simulink model "plant"  (R2026a)
settings: Solver=VariableStepAuto  StopTime=11
InitFcn:
  | run('plant_parameters.m');
values from neighbouring files (symbols this model uses):
  d = 0.1845    [plant_parameters.m]
  dd = d / sqrt(2)    [plant_parameters.m]
  Kd_J1 = 40    [plant_parameters.m]
  Kd_J2 = 30    [plant_parameters.m]
  Kd_J3 = 12    [plant_parameters.m]
  Ki_J1 = 800    [plant_parameters.m]
  Ki_J2 = 700    [plant_parameters.m]
  Ki_J3 = 300    [plant_parameters.m]
  Kp_J1 = 800    [plant_parameters.m]
  Kp_J2 = 600    [plant_parameters.m]
  Kp_J3 = 250    [plant_parameters.m]
  L1 = 0.074    [plant_parameters.m]
  L2 = 0.121    [plant_parameters.m]
  L3 = 0.230    (= 0.23)    [plant_parameters.m]
  N_J1 = 120    [plant_parameters.m]
  N_J2 = 120    [plant_parameters.m]
  N_J3 = 120    [plant_parameters.m]
  Sampling_Time = 0.005    [plant_parameters.m]
undefined symbols (not defined in the file or in its folder): X, Y, Z
libraries: sm_lib x121, nesl_utility x55, slpidlib x18
(part 8 of 8)

== matlab function plant/MATLAB Function26 ==
  data: xB_1 input; Body_X_Est output; yB_1 input; zB_1 input; xB_2 input; yB_2 input; zB_2 input; xB_3 input; yB_3 input; zB_3 input; xB_4 input; yB_4 input; zB_4 input; xB_5 input; yB_5 input; zB_5 input; xB_6 input; yB_6 input; zB_6 input; Leg1_State input; Leg2_State input; Leg3_State input; Leg4_State input; Leg5_State input; Leg6_State input; Contact6 input; Contact5 input; Contact4 input; Contact3 input; Contact2 input; Contact1 input; Body_Y_Est output; Body_Z_Est output; Valid_Leg_Count output
% Stance Contact 발의 FK 위치로 몸체 위치를 추정한다.
function [Body_X_Est, Body_Y_Est, Body_Z_Est, ...
          Valid_Leg_Count] = BodyPositionEstimator( ...
          xB_1, yB_1, zB_1, ...
          xB_2, yB_2, zB_2, ...
          xB_3, yB_3, zB_3, ...
          xB_4, yB_4, zB_4, ...
          xB_5, yB_5, zB_5, ...
          xB_6, yB_6, zB_6, ...
          Leg1_State, Leg2_State, Leg3_State, ...
          Leg4_State, Leg5_State, Leg6_State, ...
          Contact6, Contact5, Contact4, ...
          Contact3, Contact2, Contact1)

STANCE = 0;  % Stance 상태 번호를 정의한다.

persistent Initialized
persistent Body_X_Memory Body_Y_Memory Body_Z_Memory

persistent Anchor_X_1 Anchor_Y_1 Anchor_Z_1 Was_Valid_1
persistent Anchor_X_2 Anchor_Y_2 Anchor_Z_2 Was_Valid_2
persistent Anchor_X_3 Anchor_Y_3 Anchor_Z_3 Was_Valid_3
persistent Anchor_X_4 Anchor_Y_4 Anchor_Z_4 Was_Valid_4
persistent Anchor_X_5 Anchor_Y_5 Anchor_Z_5 Was_Valid_5
persistent Anchor_X_6 Anchor_Y_6 Anchor_Z_6 Was_Valid_6

% 최초 실행 시 추정 위치와 Anchor를 초기화한다.
if isempty(Initialized)
    Initialized = true;

    Body_X_Memory = 0;
    Body_Y_Memory = 0;
    Body_Z_Memory = 0;

    Anchor_X_1 = 0;
    Anchor_Y_1 = 0;
    Anchor_Z_1 = 0;
    Was_Valid_1 = false;

    Anchor_X_2 = 0;
    Anchor_Y_2 = 0;
    Anchor_Z_2 = 0;
    Was_Valid_2 = false;

    Anchor_X_3 = 0;
    Anchor_Y_3 = 0;
    Anchor_Z_3 = 0;
    Was_Valid_3 = false;

    Anchor_X_4 = 0;
    Anchor_Y_4 = 0;
    Anchor_Z_4 = 0;
    Was_Valid_4 = false;

    Anchor_X_5 = 0;
    Anchor_Y_5 = 0;
    Anchor_Z_5 = 0;
    Was_Valid_5 = false;

    Anchor_X_6 = 0;
    Anchor_Y_6 = 0;
    Anchor_Z_6 = 0;
    Was_Valid_6 = false;
end

% 1번 다리의 Anchor와 몸체 위치 후보를 계산한다.
[Anchor_X_1, Anchor_Y_1, Anchor_Z_1, Was_Valid_1, ...
 Valid_1, Body_X_1, Body_Y_1, Body_Z_1] = UpdateLegEstimate( ...
    xB_1, yB_1, zB_1, Leg1_State, Contact1, ...
    Anchor_X_1, Anchor_Y_1, Anchor_Z_1, Was_Valid_1, ...
    Body_X_Memory, Body_Y_Memory, Body_Z_Memory, STANCE);

% 2번 다리의 Anchor와 몸체 위치 후보를 계산한다.
[Anchor_X_2, Anchor_Y_2, Anchor_Z_2, Was_Valid_2, ...
 Valid_2, Body_X_2, Body_Y_2, Body_Z_2] = UpdateLegEstimate( ...
    xB_2, yB_2, zB_2, Leg2_State, Contact2, ...
    Anchor_X_2, Anchor_Y_2, Anchor_Z_2, Was_Valid_2, ...
    Body_X_Memory, Body_Y_Memory, Body_Z_Memory, STANCE);

% 3번 다리의 Anchor와 몸체 위치 후보를 계산한다.
[Anchor_X_3, Anchor_Y_3, Anchor_Z_3, Was_Valid_3, ...
 Valid_3, Body_X_3, Body_Y_3, Body_Z_3] = UpdateLegEstimate( ...
    xB_3, yB_3, zB_3, Leg3_State, Contact3, ...
    Anchor_X_3, Anchor_Y_3, Anchor_Z_3, Was_Valid_3, ...
    Body_X_Memory, Body_Y_Memory, Body_Z_Memory, STANCE);

% 4번 다리의 Anchor와 몸체 위치 후보를 계산한다.
[Anchor_X_4, Anchor_Y_4, Anchor_Z_4, Was_Valid_4, ...
 Valid_4, Body_X_4, Body_Y_4, Body_Z_4] = UpdateLegEstimate( ...
    xB_4, yB_4, zB_4, Leg4_State, Contact4, ...
    Anchor_X_4, Anchor_Y_4, Anchor_Z_4, Was_Valid_4, ...
    Body_X_Memory, Body_Y_Memory, Body_Z_Memory, STANCE);

% 5번 다리의 Anchor와 몸체 위치 후보를 계산한다.
[Anchor_X_5, Anchor_Y_5, Anchor_Z_5, Was_Valid_5, ...
 Valid_5, Body_X_5, Body_Y_5, Body_Z_5] = UpdateLegEstimate( ...
    xB_5, yB_5, zB_5, Leg5_State, Contact5, ...
    Anchor_X_5, Anchor_Y_5, Anchor_Z_5, Was_Valid_5, ...
    Body_X_Memory, Body_Y_Memory, Body_Z_Memory, STANCE);

% 6번 다리의 Anchor와 몸체 위치 후보를 계산한다.
[Anchor_X_6, Anchor_Y_6, Anchor_Z_6, Was_Valid_6, ...
 Valid_6, Body_X_6, Body_Y_6, Body_Z_6] = UpdateLegEstimate( ...
    xB_6, yB_6, zB_6, Leg6_State, Contact6, ...
    Anchor_X_6, Anchor_Y_6, Anchor_Z_6, Was_Valid_6, ...
    Body_X_Memory, Body_Y_Memory, Body_Z_Memory, STANCE);

% 현재 유효한 다리 수를 계산한다.
Valid_Leg_Count = double(Valid_1) ...
                + double(Valid_2) ...
                + double(Valid_3) ...
                + double(Valid_4) ...
                + double(Valid_5) ...
                + double(Valid_6);

% 유효 다리의 추정값을 단순 평균한다.
if Valid_Leg_Count > 0
    Body_X_Memory = (Body_X_1 + Body_X_2 + Body_X_3 ...
                   + Body_X_4 + Body_X_5 + Body_X_6) ...
                  / Valid_Leg_Count;

    Body_Y_Memory = (Body_Y_1 + Body_Y_2 + Body_Y_3 ...
                   + Body_Y_4 + Body_Y_5 + Body_Y_6) ...
                  / Valid_Leg_Count;

    Body_Z_Memory = (Body_Z_1 + Body_Z_2 + Body_Z_3 ...
                   + Body_Z_4 + Body_Z_5 + Body_Z_6) ...
                  / Valid_Leg_Count;
end

% 최종 추정 위치를 출력한다.
Body_X_Est = Body_X_Memory;
Body_Y_Est = Body_Y_Memory;
Body_Z_Est = Body_Z_Memory;

end


% 한 다리의 Anchor와 몸체 위치 후보를 계산한다.
function [Anchor_X, Anchor_Y, Anchor_Z, Was_Valid, ...
          Valid, Body_X, Body_Y, Body_Z] = UpdateLegEstimate( ...
          Foot_X, Foot_Y, Foot_Z, Leg_State, Contact, ...
          Anchor_X, Anchor_Y, Anchor_Z, Was_Valid, ...
          Body_X_Previous, Body_Y_Previous, Body_Z_Previous, ...
          Stance_State)

% Stance이면서 접촉 중인 다리만 유효하게 사용한다.
Valid = (Leg_State == Stance_State) && (Contact ~= 0);

% 새로 유효해진 순간에 발의 기준 좌표계 Anchor를 저장한다.
if Valid && ~Was_Valid
    Anchor_X = Body_X_Previous + Foot_X;
    Anchor_Y = Body_Y_Previous + Foot_Y;
    Anchor_Z = Body_Z_Previous + Foot_Z;
end

% 유효 다리는 Anchor와 현재 FK 위치로 몸체 위치를 계산한다.
if Valid
    Body_X = Anchor_X - Foot_X;
    Body_Y = Anchor_Y - Foot_Y;
    Body_Z = Anchor_Z - Foot_Z;
else
    Body_X = 0;
    Body_Y = 0;
    Body_Z = 0;
end

Was_Valid = Valid;

end

== matlab function plant/Plant/MATLAB Function1 ==
  data: t input; Contact1 output; Contact2 output; Contact3 output; Contact4 output; Contact5 output; Contact6 output
% 모든 다리에 강한 Early 및 Late Landing 시험 신호를 생성한다.
function [Contact1, Contact2, Contact3, ...
          Contact4, Contact5, Contact6] = TestContact(t)

Gait_Start_Time = 1.0;  % 보행 시작 시간을 정의한다.
Pattern_Time    = 7.18; % 12개 시험 Phase의 전체 시간을 정의한다.

% 보행 시작 전에는 모든 발을 접촉 상태로 둔다.
Contact1 = 1;
Contact2 = 1;
Contact3 = 1;
Contact4 = 1;
Contact5 = 1;
Contact6 = 1;

if t < Gait_Start_Time
    return;
end

% 반복 패턴 내부의 현재 시간을 계산한다.
elapsed_time = t - Gait_Start_Time;
cycle_count  = floor(elapsed_time/Pattern_Time);
cycle_time   = elapsed_time - cycle_count*Pattern_Time;

% Late Landing 지연을 포함한 현재 시험 Phase를 선택한다.
if cycle_time < 0.59
    phase_pattern = 0;
    phase_time    = cycle_time;
elseif cycle_time < 1.20
    phase_pattern = 1;
    phase_time    = cycle_time - 0.59;
elseif cycle_time < 1.78
    phase_pattern = 2;
    phase_time    = cycle_time - 1.20;
elseif cycle_time < 2.38
    phase_pattern = 3;
    phase_time    = cycle_time - 1.78;
elseif cycle_time < 3.00
    phase_pattern = 4;
    phase_time    = cycle_time - 2.38;
elseif cycle_time < 3.59
    phase_pattern = 5;
    phase_time    = cycle_time - 3.00;
elseif cycle_time < 4.20
    phase_pattern = 6;
    phase_time    = cycle_time - 3.59;
elseif cycle_time < 4.77
    phase_pattern = 7;
    phase_time    = cycle_time - 4.20;
elseif cycle_time < 5.37
    phase_pattern = 8;
    phase_time    = cycle_time - 4.77;
elseif cycle_time < 5.99
    phase_pattern = 9;
    phase_time    = cycle_time - 5.37;
elseif cycle_time < 6.57
    phase_pattern = 10;
    phase_time    = cycle_time - 5.99;
else
    phase_pattern = 11;
    phase_time    = cycle_time - 6.57;
end

% Phase마다 세 Swing 다리의 접촉 시점을 다르게 설정한다.
switch phase_pattern
    case 0
        landing_1 = 0.34;
        landing_2 = 0.50;
        landing_3 = 0.59;
    case 1
        landing_1 = 0.61;
        landing_2 = 0.37;
        landing_3 = 0.50;
    case 2
        landing_1 = 0.50;
        landing_2 = 0.39;
        landing_3 = 0.58;
    case 3
        landing_1 = 0.33;
        landing_2 = 0.60;
        landing_3 = 0.50;
    case 4
        landing_1 = 0.62;
        landing_2 = 0.50;
        landing_3 = 0.36;
    case 5
        landing_1 = 0.50;
        landing_2 = 0.40;
        landing_3 = 0.59;
    case 6
        landing_1 = 0.38;
        landing_2 = 0.61;
        landing_3 = 0.50;
    case 7
        landing_1 = 0.57;
        landing_2 = 0.50;
        landing_3 = 0.35;
    case 8
        landing_1 = 0.50;
        landing_2 = 0.34;
        landing_3 = 0.60;
    case 9
        landing_1 = 0.39;
        landing_2 = 0.62;
        landing_3 = 0.50;
    case 10
        landing_1 = 0.58;
        landing_2 = 0.50;
        landing_3 = 0.33;
    otherwise
        landing_1 = 0.50;
        landing_2 = 0.36;
        landing_3 = 0.61;
end

% 짝수 Phase에서는 1, 3, 5번 다리에 접촉 시험을 적용한다.
if mod(phase_pattern, 2) == 0
    Contact1 = double(phase_time >= landing_1);
    Contact3 = double(phase_time >= landing_2);
    Contact5 = double(phase_time >= landing_3);

% 홀수 Phase에서는 2, 4, 6번 다리에 접촉 시험을 적용한다.
else
    Contact2 = double(phase_time >= landing_1);
    Contact4 = double(phase_time >= landing_2);
    Contact6 = double(phase_time >= landing_3);
end

end

== matlab function plant/MATLAB Function1 ==
  data: xL output; yL output; q1 input; q2 input; q3 input; zL output
function [xL, yL, zL] = legFK(q1, q2, q3)
% 현재 관절각으로 발끝 위치를 계산한다.

L1 = 0.074;   % 링크1 에서 링크1 까지 거리 (m)
L2 = 0.121;   % 링크2 에서 링크3 까지 거리 (m)
L3 = 0.230;   % 링크3 에서 발 끝 까지 거리 (m)

r = L1 + L2*cos(q2) + L3*cos(q2 + q3);    % 수평 도달 거리를 계산한다.

xL = r*cos(q1);                            % 다리 좌표계 x 위치를 계산한다.
yL = r*sin(q1);                            % 다리 좌표계 y 위치를 계산한다.
zL = -L2*sin(q2) - L3*sin(q2 + q3);        % 다리 좌표계 z 위치를 계산한다.
end

== matlab function plant/MATLAB Function ==
  data: vx input; vy input; vz input; wx input; wy input; wz input; xB_1 output; yB_1 output; zB_1 output; xB_2 output; yB_2 output; zB_2 output; xB_3 output; yB_3 output; zB_3 output; xB_4 output; yB_4 output; zB_4 output; xB_5 output; yB_5 output; zB_5 output; xB_6 output; yB_6 output; zB_6 output; Leg1_State input; Leg1_Progress input; Leg2_State input; Leg2_Progress input; Leg3_State input; Leg3_Progress input; Leg4_State input; Leg4_Progress input; Leg5_State input; Leg5_Progress input; Leg6_State input; Leg6_Progress input; Startup_Phase input
% 다리별 보행 상태와 Body Twist로 6개 발 목표를 생성한다.
function [xB_1, yB_1, zB_1, ...
          xB_2, yB_2, zB_2, ...
          xB_3, yB_3, zB_3, ...
          xB_4, yB_4, zB_4, ...
          xB_5, yB_5, zB_5, ...
          xB_6, yB_6, zB_6] = ...
    TripodFootTrajectory( ...
          vx, vy, vz, wx, wy, wz, ...
          Leg1_State, Leg1_Progress, ...
          Leg2_State, Leg2_Progress, ...
          Leg3_State, Leg3_Progress, ...
          Leg4_State, Leg4_Progress, ...
          Leg5_State, Leg5_Progress, ...
          Leg6_State, Leg6_Progress, ...
          Startup_Phase)

STANCE       = 0;  % Stance 상태 번호를 정의한다.
SWING        = 1;  % Swing 상태 번호를 정의한다.
LATE_LANDING = 2;  % Late Landing 상태 번호를 정의한다.

Sampling_Time       = 0.005; % 제어 주기를 정의한다.
Phase_Time          = 0.5;   % 한 Tripod Phase 시간을 정의한다.
Swing_Height        = 0.20;  % Swing 발의 최대 상승 높이를 정의한다. (범위: 20cm -+5cm)
Swing_Radial_Offset = 0.07;  % Swing 중간점의 바깥쪽 이동량을 정의한다.
Search_Speed        = 0.2;  % Late Landing 하강 속도를 정의한다.
Early_Min_Progress  = 0.5;   % Early Landing 판정 시작점을 정의한다.

% 다리별 장착 방향을 정의한다.
alpha_1 = -pi/4;
alpha_2 = -pi/2;
alpha_3 = -3*pi/4;
alpha_4 =  pi/4;
alpha_5 =  pi/2;
alpha_6 =  3*pi/4;

% 로봇 형상값을 정의한다.
d  = 0.1845;
dd = d/sqrt(2);

L1 = 0.074;
L2 = 0.121;
L3 = 0.230;

% 초기 관절각을 정의한다.
q2_init = 30*pi/180;
q3_init = 50*pi/180;

% 초기 Leg 좌표를 계산한다.
xL0 = L1 + L2*cos(q2_init) + L3*cos(q2_init + q3_init);
zL0 = -L2*sin(q2_init) - L3*sin(q2_init + q3_init);
c45 = cos(pi/4);

% 1번 다리 초기 Body 좌표를 계산한다.
x0_1 =  dd + c45*xL0;
y0_1 = -dd - c45*xL0;
z0_1 =  zL0;

% 2번 다리 초기 Body 좌표를 계산한다.
x0_2 = 0;
y0_2 = -d - xL0;
z0_2 = zL0;

% 3번 다리 초기 Body 좌표를 계산한다.
x0_3 = -dd - c45*xL0;
y0_3 = -dd - c45*xL0;
z0_3 =  zL0;

% 4번 다리 초기 Body 좌표를 계산한다.
x0_4 = dd + c45*xL0;
y0_4 = dd + c45*xL0;
z0_4 = zL0;

% 5번 다리 초기 Body 좌표를 계산한다.
x0_5 = 0;
y0_5 = d + xL0;
z0_5 = zL0;

% 6번 다리 초기 Body 좌표를 계산한다.
x0_6 = -dd - c45*xL0;
y0_6 =  dd + c45*xL0;
z0_6 =  zL0;

% 1번 다리의 한 Phase 동안 Stance 이동량을 계산한다.
dx_1 = Phase_Time*(-vx - wy*z0_1 + wz*y0_1);
dy_1 = Phase_Time*(-vy - wz*x0_1 + wx*z0_1);
dz_1 = Phase_Time*(-vz - wx*y0_1 + wy*x0_1);

% 2번 다리의 한 Phase 동안 Stance 이동량을 계산한다.
dx_2 = Phase_Time*(-vx - wy*z0_2 + wz*y0_2);
dy_2 = Phase_Time*(-vy - wz*x0_2 + wx*z0_2);
dz_2 = Phase_Time*(-vz - wx*y0_2 + wy*x0_2);

% 3번 다리의 한 Phase 동안 Stance 이동량을 계산한다.
dx_3 = Phase_Time*(-vx - wy*z0_3 + wz*y0_3);
dy_3 = Phase_Time*(-vy - wz*x0_3 + wx*z0_3);
dz_3 = Phase_Time*(-vz - wx*y0_3 + wy*x0_3);

% 4번 다리의 한 Phase 동안 Stance 이동량을 계산한다.
dx_4 = Phase_Time*(-vx - wy*z0_4 + wz*y0_4);
dy_4 = Phase_Time*(-vy - wz*x0_4 + wx*z0_4);
dz_4 = Phase_Time*(-vz - wx*y0_4 + wy*x0_4);

% 5번 다리의 한 Phase 동안 Stance 이동량을 계산한다.
dx_5 = Phase_Time*(-vx - wy*z0_5 + wz*y0_5);
dy_5 = Phase_Time*(-vy - wz*x0_5 + wx*z0_5);
dz_5 = Phase_Time*(-vz - wx*y0_5 + wy*x0_5);

% 6번 다리의 한 Phase 동안 Stance 이동량을 계산한다.
dx_6 = Phase_Time*(-vx - wy*z0_6 + wz*y0_6);
dy_6 = Phase_Time*(-vy - wz*x0_6 + wx*z0_6);
dz_6 = Phase_Time*(-vz - wx*y0_6 + wy*x0_6);

% 1번 다리의 최종 발 목표를 계산한다.
[xB_1, yB_1, zB_1] = AdaptiveFootTarget( ...
    1, Leg1_State, Leg1_Progress, Startup_Phase, ...
    x0_1, y0_1, z0_1, dx_1, dy_1, dz_1, alpha_1, ...
    vx, vy, vz, wx, wy, wz, Sampling_Time, ...
    Swing_Height, Swing_Radial_Offset, Search_Speed, ...
    Early_Min_Progress, STANCE, SWING, LATE_LANDING);

% 2번 다리의 최종 발 목표를 계산한다.
[xB_2, yB_2, zB_2] = AdaptiveFootTarget( ...
    2, Leg2_State, Leg2_Progress, Startup_Phase, ...
    x0_2, y0_2, z0_2, dx_2, dy_2, dz_2, alpha_2, ...
    vx, vy, vz, wx, wy, wz, Sampling_Time, ...
    Swing_Height, Swing_Radial_Offset, Search_Speed, ...
    Early_Min_Progress, STANCE, SWING, LATE_LANDING);

% 3번 다리의 최종 발 목표를 계산한다.
[xB_3, yB_3, zB_3] = AdaptiveFootTarget( ...
    3, Leg3_State, Leg3_Progress, Startup_Phase, ...
    x0_3, y0_3, z0_3, dx_3, dy_3, dz_3, alpha_3, ...
    vx, vy, vz, wx, wy, wz, Sampling_Time, ...
    Swing_Height, Swing_Radial_Offset, Search_Speed, ...
    Early_Min_Progress, STANCE, SWING, LATE_LANDING);

% 4번 다리의 최종 발 목표를 계산한다.
[xB_4, yB_4, zB_4] = AdaptiveFootTarget( ...
    4, Leg4_State, Leg4_Progress, Startup_Phase, ...
    x0_4, y0_4, z0_4, dx_4, dy_4, dz_4, alpha_4, ...
    vx, vy, vz, wx, wy, wz, Sampling_Time, ...
    Swing_Height, Swing_Radial_Offset, Search_Speed, ...
    Early_Min_Progress, STANCE, SWING, LATE_LANDING);

% 5번 다리의 최종 발 목표를 계산한다.
[xB_5, yB_5, zB_5] = AdaptiveFootTarget( ...
    5, Leg5_State, Leg5_Progress, Startup_Phase, ...
    x0_5, y0_5, z0_5, dx_5, dy_5, dz_5, alpha_5, ...
    vx, vy, vz, wx, wy, wz, Sampling_Time, ...
    Swing_Height, Swing_Radial_Offset, Search_Speed, ...
    Early_Min_Progress, STANCE, SWING, LATE_LANDING);

% 6번 다리의 최종 발 목표를 계산한다.
[xB_6, yB_6, zB_6] = AdaptiveFootTarget( ...
    6, Leg6_State, Leg6_Progress, Startup_Phase, ...
    x0_6, y0_6, z0_6, dx_6, dy_6, dz_6, alpha_6, ...
    vx, vy, vz, wx, wy, wz, Sampling_Time, ...
    Swing_Height, Swing_Radial_Offset, Search_Speed, ...
    Early_Min_Progress, STANCE, SWING, LATE_LANDING);

end


% 접촉 상태에 맞춰 한 다리의 최종 발 목표를 계산한다.
function [x, y, z] = AdaptiveFootTarget( ...
    leg_id, leg_state, progress, startup_phase, ...
    x0, y0, z0, dx, dy, dz, leg_angle, ...
    vx, vy, vz, wx, wy, wz, sampling_time, ...
    swing_height, radial_offset, search_speed, ...
    early_min_progress, stance_state, swing_state, late_state)

persistent Initialized X_Memory Y_Memory Z_Memory Previous_State
persistent Adapted_Stance Custom_Swing
persistent Swing_Start_X Swing_Start_Y Swing_Start_Z

if isempty(Initialized)
    Initialized     = true;
    X_Memory        = zeros(1, 6);
    Y_Memory        = zeros(1, 6);
    Z_Memory        = zeros(1, 6);
    Previous_State  = zeros(1, 6);
    Adapted_Stance  = false(1, 6);
    Custom_Swing    = false(1, 6);
    Swing_Start_X   = zeros(1, 6);
    Swing_Start_Y   = zeros(1, 6);
    Swing_Start_Z   = zeros(1, 6);
end

i = leg_id;

% 중립점을 기준으로 앞쪽과 뒤쪽 끝점을 계산한다.
x_front = x0 - 0.5*dx;
y_front = y0 - 0.5*dy;
z_front = z0 - 0.5*dz;

x_rear = x0 + 0.5*dx;
y_rear = y0 + 0.5*dy;
z_rear = z0 + 0.5*dz;

% 현재 Phase의 기본 Swing 시작점을 선택한다.
if startup_phase
    x_swing_start = x0;
    y_swing_start = y0;
    z_swing_start = z0;
else
    x_swing_start = x_rear;
    y_swing_start = y_rear;
    z_swing_start = z_rear;
end

% Late Landing에서는 착지 끝점부터 아래쪽으로 탐색한다.
if leg_state == late_state
    if Previous_State(i) ~= late_state
        [X_Memory(i), Y_Memory(i), Z_Memory(i)] = SwingTarget( ...
            1, ...
            x_swing_start, y_swing_start, z_swing_start, ...
            x_front, y_front, z_front, ...
            swing_height, radial_offset, leg_angle);
    else
        Search_Inward_Ratio = 0.8;  % 하강 속도 대비 안쪽 이동 비율을 정의한다.
        inward_speed = Search_Inward_Ratio*search_speed;

        X_Memory(i) = X_Memory(i) ...
                    - inward_speed*cos(leg_angle)*sampling_time;

        Y_Memory(i) = Y_Memory(i) ...
                    - inward_speed*sin(leg_angle)*sampling_time;

        Z_Memory(i) = Z_Memory(i) ...
                    - search_speed*sampling_time;
    end

    Adapted_Stance(i) = true;

    x = X_Memory(i);
    y = Y_Memory(i);
    z = Z_Memory(i);

% Swing에서는 저장된 실제 이륙점 또는 기본 끝점을 사용한다.
elseif leg_state == swing_state
    if Previous_State(i) ~= swing_state
        if Adapted_Stance(i)
            Swing_Start_X(i) = X_Memory(i);
            Swing_Start_Y(i) = Y_Memory(i);
            Swing_Start_Z(i) = Z_Memory(i);
            Custom_Swing(i)  = true;
        else
            Swing_Start_X(i) = x_swing_start;
            Swing_Start_Y(i) = y_swing_start;
            Swing_Start_Z(i) = z_swing_start;
            Custom_Swing(i)  = false;
        end

        Adapted_Stance(i) = false;
    end

    if Custom_Swing(i)
        x_swing_start = Swing_Start_X(i);
        y_swing_start = Swing_Start_Y(i);
        z_swing_start = Swing_Start_Z(i);
    end

    [x, y, z] = SwingTarget( ...
        progress, ...
        x_swing_start, y_swing_start, z_swing_start, ...
        x_front, y_front, z_front, ...
        swing_height, radial_offset, leg_angle);

    X_Memory(i) = x;
    Y_Memory(i) = y;
    Z_Memory(i) = z;

% Early 또는 Late Landing 이후에는 저장 위치에서 Stance를 계속한다.
elseif leg_state == stance_state
    if Previous_State(i) == late_state
        Adapted_Stance(i) = true;

    elseif Previous_State(i) == swing_state && ...
            progress >= early_min_progress

        if Custom_Swing(i)
            x_swing_start = Swing_Start_X(i);
            y_swing_start = Swing_Start_Y(i);
            z_swing_start = Swing_Start_Z(i);
        end

        [X_Memory(i), Y_Memory(i), Z_Memory(i)] = SwingTarget( ...
            progress, ...
            x_swing_start, y_swing_start, z_swing_start, ...
            x_front, y_front, z_front, ...
            swing_height, radial_offset, leg_angle);

        Adapted_Stance(i) = true;

    elseif Adapted_Stance(i)
        x_dot = -vx - wy*Z_Memory(i) + wz*Y_Memory(i);
        y_dot = -vy - wz*X_Memory(i) + wx*Z_Memory(i);
        z_dot = -vz - wx*Y_Memory(i) + wy*X_Memory(i);

        X_Memory(i) = X_Memory(i) + x_dot*sampling_time;
        Y_Memory(i) = Y_Memory(i) + y_dot*sampling_time;
        Z_Memory(i) = Z_Memory(i) + z_dot*sampling_time;

    elseif startup_phase
        [X_Memory(i), Y_Memory(i), Z_Memory(i)] = StanceTarget( ...
            progress, ...
            x0, y0, z0, ...
            x_rear, y_rear, z_rear);

    else
        [X_Memory(i), Y_Memory(i), Z_Memory(i)] = StanceTarget( ...
            progress, ...
            x_front, y_front, z_front, ...
            x_rear, y_rear, z_rear);
    end

    x = X_Memory(i);
    y = Y_Memory(i);
    z = Z_Memory(i);

% 정의되지 않은 상태에서는 직전 목표를 유지한다.
else
    x = X_Memory(i);
    y = Y_Memory(i);
    z = Z_Memory(i);
end

Previous_State(i) = leg_state;

end


% Quintic과 Cubic Bezier로 Swing 발 목표를 계산한다.
function [x, y, z] = SwingTarget( ...
    progress, ...
    x_start, y_start, z_start, ...
    x_end, y_end, z_end, ...
    swing_height, radial_offset, leg_angle)

% 진행률을 0~1 범위로 제한한다.
if progress < 0
    progress = 0;
elseif progress > 1
    progress = 1;
end

% Quintic Time Scaling을 계산한다.
s = 10*progress^3 ...
  - 15*progress^4 ...
  + 6*progress^5;

% 최고 높이가 설정값과 일치하도록 제어점을 계산한다.
bezier_height = (4/3)*swing_height;

z_control_1 = z_start + bezier_height;
z_control_2 = z_end   + bezier_height;

% Cubic Bezier 계수를 계산한다.
one_minus_s = 1 - s;

b0 = one_minus_s^3;
b1 = 3*one_minus_s^2*s;
b2 = 3*one_minus_s*s^2;
b3 = s^3;

% Swing 발 목표를 계산한다.
x = b0*x_start ...
  + b1*x_start ...
  + b2*x_end ...
  + b3*x_end;

y = b0*y_start ...
  + b1*y_start ...
  + b2*y_end ...
  + b3*y_end;

z = b0*z_start ...
  + b1*z_control_1 ...
  + b2*z_control_2 ...
  + b3*z_end;

% Swing 중간점에서 발을 다리 바깥쪽으로 이동한다.
radial_bulge = radial_offset*4*s*(1-s);

x = x + radial_bulge*cos(leg_angle);
y = y + radial_bulge*sin(leg_angle);

end


% 선형 보간으로 Stance 발 목표를 계산한다.
function [x, y, z] = StanceTarget( ...
    progress, ...
    x_start, y_start, z_start, ...
    x_end, y_end, z_end)

% 진행률을 0~1 범위로 제한한다.
if progress < 0
    progress = 0;
elseif progress > 1
    progress = 1;
end

% Stance 발 목표를 계산한다.
x = x_start + progress*(x_end - x_start);
y = y_start + progress*(y_end - y_start);
z = z_start + progress*(z_end - z_start);

end
